simulink model "MPC"  (R2018a)
settings: Solver=VariableStepAuto  StartTime=0.0  StopTime=10  RelTol=1e-3
PreLoadFcn:
  | modelDir = fileparts(get_param(bdroot, 'FileName'));
  | addpath(modelDir);
  | addpath(fullfile(modelDir,'../../Parameters'));
  | addpath(fullfile(modelDir,'../../Controllers/MPC'));
  | addpath(fullfile(modelDir,'../../Controllers/MPC/functions'));
  | addpath(fullfile(modelDir,'../../Controllers/MPC/functions/polynomial'));
  | addpath(fullfile(modelDir,'../../Controllers/MPC/functions/trajectory'));
  | addpath(fullfile(modelDir,'../../Controllers/MPC/functions/visualization'));
  | addpath(fullfile(modelDir,'../../Controllers/MPC/generated'));
  | addpath(fullfile(modelDir,'../../Misc'));
  | 
  | Parameters_Controllers % for controller sample rate
  | Parameters_Simulation
  | Constants_Kugle
  | Constants_nominal
  | Parameters_MPC;
  | 
  | PrepareMPCtrajectory;
InitFcn:
  | Parameters_Controllers % for controller sample rate
  | Parameters_Simulation
  | Constants_Kugle
  | Constants_nominal
  | Parameters_MPC;
  | 
  | close all; % close opened plots to prepare for automatic plots for MPC visualization
  | 
  | PrepareMPCtrajectory;
values from neighbouring files (symbols this model uses):
  MPC_Obstacles = [MPC_Obstacles; repmat([100, 100, 1], [(5-size(MPC_Obstacles,1)),1])]    [PrepareMPCtrajectory.m]
undefined symbols (not defined in the file or in its folder): maxAngle, maxdOmegaRef, maxOmegaRef, maxVelocity, minVelocity, MPC_DesiredVelocity, MPC_HeadingAngularVelocity, MPC_Trajectory, MPC_u0, MPC_x0, N, pathApproximationOrder, ProximityOffset, ProximityScale, Ts, Ts_MPC, WindowHeight, WindowOffset, WindowOrientationSelection, WindowWidth, Wmat, WNmat, x_init
libraries: qlib x1
settings Model: Creator=Thomas  LastModifiedBy=Thomas
settings DataIOCC: SaveOutput=off  SignalLogging=off  DSMLogging=off
settings ModelReferenceCC: ModelReferenceNumInstancesAllowed=Single  ModelReferencePassRootInputsByReference=off  ModelReferenceMinAlgLoopOccurrences=on

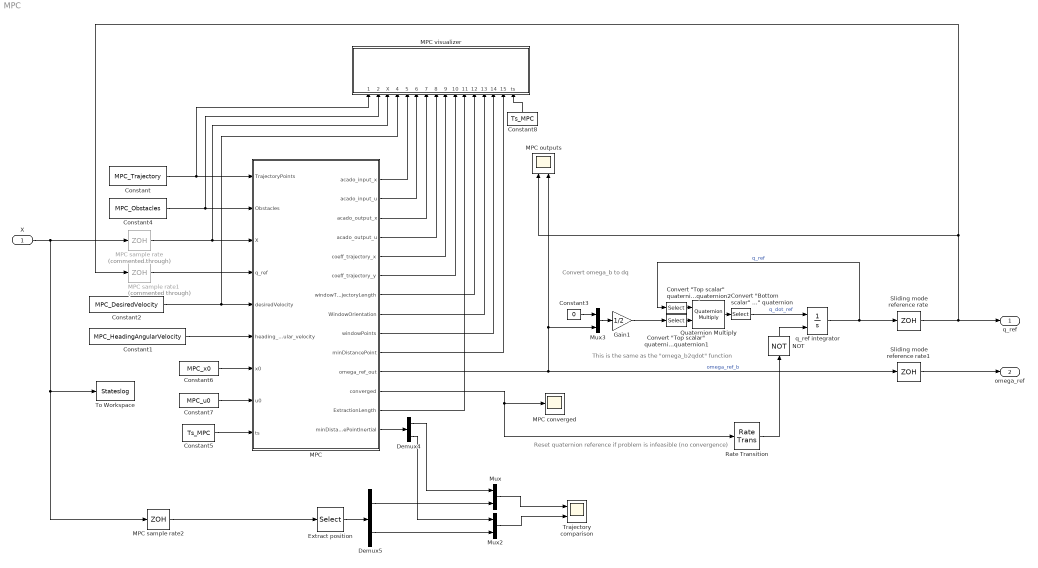
== system MPC ==
  note: Reset quaternion reference if problem is infeasible (no convergence)
  note: This is the same as the "omega_b2qdot" function
  note: Convert omega_b to dq
  X : Inport  PortDimensions=12
  Constant : Constant  Value=MPC_Trajectory  SampleTime=-1
  Constant1 : Constant  Value=MPC_HeadingAngularVelocity  SampleTime=-1
  Constant2 : Constant  Value=MPC_DesiredVelocity  SampleTime=-1
  Constant3 : Constant  Value=0
  Constant4 : Constant  Value=MPC_Obstacles  SampleTime=-1
  Constant5 : Constant  Value=Ts_MPC  SampleTime=-1
  Constant6 : Constant  Value=MPC_x0  SampleTime=-1
  Constant7 : Constant  Value=MPC_u0  SampleTime=-1
  Constant8 : Constant  Value=Ts_MPC  SampleTime=Ts_MPC
  "Convert \"Bottom scalar\" quaternion to \"Top scalar\" quaternion" : Selector  InputPortWidth=4  IndexOptions=Index vector (dialog)  Indices=[4 1 2 3]  OutputSizes=1
  "Convert \"Top scalar\" quaternion to \"Bottom scalar\" quaternion1" : Selector  InputPortWidth=4  IndexOptions=Index vector (dialog)  Indices=[2 3 4 1]  OutputSizes=1
  "Convert \"Top scalar\" quaternion to \"Bottom scalar\" quaternion2" : Selector  InputPortWidth=4  IndexOptions=Index vector (dialog)  Indices=[2 3 4 1]  OutputSizes=1
  Demux4 : Demux  Outputs=2
  Demux5 : Demux  Outputs=2
  Extract position : Selector  InputPortWidth=12  IndexOptions=Index vector (dialog)  Indices=[1 2]  OutputSizes=1
  Gain1 : Gain  Gain=1/2
  MPC : MATLAB Function  TreatAsAtomicUnit=on  SystemSampleTime=Ts_MPC
      settings: MinAlgLoopOccurrences=on
  MPC converged : Scope
  MPC outputs : Scope  NumInputPorts=2
  MPC sample rate : ZeroOrderHold  Commented=through  SampleTime=Ts_MPC
  MPC sample rate1 : ZeroOrderHold  Commented=through  SampleTime=Ts_MPC
  MPC sample rate2 : ZeroOrderHold  SampleTime=Ts_MPC
  MPC visualizer : MATLAB Function  TreatAsAtomicUnit=on  SystemSampleTime=Ts_MPC
      settings: MinAlgLoopOccurrences=on
  Mux : Mux  Inputs=2
  Mux2 : Mux  Inputs=2
  Mux3 : Mux  Inputs=2
  NOT : Logic  Operator=NOT  IconShape=distinctive  AllPortsSameDT=off  OutDataTypeStr=boolean
  Quaternion Multiply : qlib/Quaternion Multiply
  Rate Transition : RateTransition
  Sliding mode reference rate : ZeroOrderHold  SampleTime=Ts
  Sliding mode reference rate1 : ZeroOrderHold  SampleTime=Ts
  To Workspace : ToWorkspace  VariableName=Stateslog  SaveFormat=Timeseries  SampleTime=-1
  Trajectory comparison : Scope  NumInputPorts=2
  q_ref integrator : Integrator  ExternalReset=level hold  InitialCondition=x_init(3:6)
  q_ref : Outport  PortDimensions=4
  omega_ref : Outport  Port=2  PortDimensions=3
  wires:
  X/1 -> MPC sample rate/1, MPC sample rate2/1, To Workspace/1
  MPC/5(coeff_trajectory_x) -> MPC visualizer/9(coeff_trajectory_x)
  Constant2/1 -> MPC visualizer/4(velocity), MPC/5(desiredVelocity)
  Mux/1 -> Trajectory comparison/1
  MPC/10(minDistancePoint) -> MPC visualizer/15(minDistancePoint)
  MPC/14(minDistancePointInertial) -> Demux4/1
  Demux5/2 -> Mux2/2
  MPC/2(acado_input_u) -> MPC visualizer/6(acado_input_u)
  Demux5/1 -> Mux/2
  MPC sample rate/1 -> MPC visualizer/3(X), MPC/3(X)
  Mux2/1 -> Trajectory comparison/2
  Extract position/1 -> Demux5/1
  Demux4/2 -> Mux2/1
  MPC/6(coeff_trajectory_y) -> MPC visualizer/10(coeff_trajectory_y)
  Sliding mode reference rate/1 -> MPC sample rate1/1, MPC outputs/1, q_ref/1
  "Convert \"Bottom scalar\" quaternion to \"Top scalar\" quaternion"/1 -> q_ref integrator/1  "q_dot_ref"
  Demux4/1 -> Mux/1
  MPC sample rate1/1 -> MPC/4(q_ref)
  Constant/1 -> MPC visualizer/1(TrajectoryPoints), MPC/1(TrajectoryPoints)
  q_ref integrator/1 -> "Convert \"Top scalar\" quaternion to \"Bottom scalar\" quaternion2"/1, Sliding mode reference rate/1  "q_ref"
  MPC/1(acado_input_x) -> MPC visualizer/5(acado_input_x)
  MPC/8(WindowOrientation) -> MPC visualizer/13(WindowOrientation)
  MPC/4(acado_output_u) -> MPC visualizer/8(acado_output_u)
  MPC/3(acado_output_x) -> MPC visualizer/7(acado_output_x)
  MPC/7(windowTrajectoryLength) -> MPC visualizer/12(trajectoryLength)
  "Convert \"Top scalar\" quaternion to \"Bottom scalar\" quaternion1"/1 -> Quaternion Multiply/2
  Gain1/1 -> "Convert \"Top scalar\" quaternion to \"Bottom scalar\" quaternion1"/1
  "Convert \"Top scalar\" quaternion to \"Bottom scalar\" quaternion2"/1 -> Quaternion Multiply/1
  Mux3/1 -> Gain1/1
  Constant3/1 -> Mux3/1
  Quaternion Multiply/1 -> "Convert \"Bottom scalar\" quaternion to \"Top scalar\" quaternion"/1
  MPC/11(omega_ref_out) -> Sliding mode reference rate1/1, MPC outputs/2, Mux3/2  "omega_ref_b"
  Constant1/1 -> MPC/6(heading_angular_velocity)
  Constant5/1 -> MPC/9(ts)
  Constant4/1 -> MPC visualizer/2(Obstacles), MPC/2(Obstacles)
  Sliding mode reference rate1/1 -> omega_ref/1
  MPC sample rate2/1 -> Extract position/1
  Constant6/1 -> MPC/7(x0)
  Constant7/1 -> MPC/8(u0)
  MPC/13(ExtractionLength) -> MPC visualizer/11(ExtractionLength)
  Constant8/1 -> MPC visualizer/16(ts)
  MPC/9(windowPoints) -> MPC visualizer/14(windowPoints)
  NOT/1 -> q_ref integrator/2
  MPC/12(converged) -> Rate Transition/1, MPC converged/1
  Rate Transition/1 -> NOT/1

== matlab function MPC/MPC ==
  data: TrajectoryPoints input; Obstacles input; X input size=12; q_ref input size=4; desiredVelocity input; heading_angular_velocity input; N parameter; x0 input size=[1,length(MPC_x0)]; u0 input size=[1,length(MPC_u0)]; acado_input_x output size=[N+1,length(MPC_x0)]; acado_input_u output size=[N,length(MPC_u0)]; acado_output_x output size=[N+1,length(MPC_x0)]; acado_output_u output size=[N,length(MPC_u0)]; coeff_trajectory_x output size=[10,1]; coeff_trajectory_y output size=[10,1]; windowTrajectoryLength output; WindowOrientation output; windowPoints output size=[100,2]; minDistancePoint output; omega_ref_out output; converged output; ExtractionLength output; minDistancePointInertial output; pathApproximationOrder parameter; WindowOrientationSelection parameter; minVelocity parameter; maxOmegaRef parameter; maxAngle parameter; WNmat parameter; Wmat parameter; ts input; maxVelocity parameter; maxdOmegaRef parameter; ProximityOffset parameter; ProximityScale parameter
function [acado_input_x, acado_input_u, acado_output_x, acado_output_u, coeff_trajectory_x, coeff_trajectory_y, windowTrajectoryLength, WindowOrientation, windowPoints, minDistancePoint, omega_ref_out, converged, ExtractionLength, minDistancePointInertial] = MPC(TrajectoryPoints, Obstacles, X, q_ref, desiredVelocity, heading_angular_velocity, N, x0, u0, pathApproximationOrder, WindowOrientationSelection, minVelocity, maxOmegaRef, maxAngle, WNmat, Wmat, ts, maxVelocity, maxdOmegaRef, ProximityOffset, ProximityScale)
    Phi = @(q)[q(1) -q(2) -q(3) -q(4);     % for q o p = Phi(q) * p
              q(2) q(1)  -q(4) q(3);
              q(3) q(4)  q(1)  -q(2);
              q(4) -q(3) q(2)  q(1)];           
    Gamma = @(p)[p(1) -p(2) -p(3) -p(4);   % for q o p = Gamma(p) * q
                 p(2) p(1) p(4) -p(3);
                 p(3) -p(4) p(1) p(2);
                 p(4) p(3) -p(2) p(1)];  

    devec = [0,1,0,0;0,0,1,0;0,0,0,1]; % 'v' in notes
    vec = [0,0,0;1,0,0;0,1,0;0,0,1]; % '^' in notes
   
    x = X(1);
    y = X(2);
    q1 = X(3);
    q2 = X(4);
    q3 = X(5);
    q4 = X(6);
    q = [q1,q2,q3,q4]';
   
    % OBS! It seems to be quite important to use the filtered translational velocity which does not have spikes due to changes in the attitude
    dx = X(7);
    dy = X(8);
    dq1 = X(9);
    dq2 = X(10);
    dq3 = X(11);
    dq4 = X(12);      
        
    coder.extrinsic('ExtractWindowTrajectory_mex');
    coder.extrinsic('ExtractDistanceTrajectory_mex');
    coder.extrinsic('kugle_mpc_obstacles');
    
    % Convert states for MPC abstraction (robot-centric frame - Ferret frame???)      
    ResetAtConvergenceProblems = false;
    UseCurrentQuaternionAsReference = false; % if set to true, the current system state will be used at each iteration to define the current quaternion
    if (~UseCurrentQuaternionAsReference)
        q = q_ref;
    end    
    
    % Extract current robot yaw (heading)
    p = Phi(q)*Gamma(q)'*[0,1,0,0]';
    RobotYaw = atan2(p(3),p(2));   
    q_heading = [cos(RobotYaw/2);0;0;sin(RobotYaw/2)];
    q_tilt = Phi(q_heading)' * q; % tilt in heading frame    
    if (q_tilt(1) < 0)
        q_tilt = -q_tilt; % invert q_tilt to take shortest rotation
    end
    R_heading = [cos(RobotYaw), sin(RobotYaw);
                 -sin(RobotYaw), cos(RobotYaw)];                   
           
    persistent PreviousHorizonLength;
    if (isempty(PreviousHorizonLength))   
        PreviousHorizonLength = 0;
    end

    persistent xInit; 
    if (isempty(xInit))   
        fprintf('Initializing MPC\n');
        %xInit = zeros(N+1, length(x0));        
        xInit = repmat(x0, [(N+1),1]);
        %xInit(:,7) = ts * desiredVelocity * (0:N)'; % generate increasing S init values based on desired velocity
        %xInit(:,8) = repmat(desiredVelocity, [N+1, 1]); % set ds to desired velocity when initializing
    end    
    persistent uInit; 
    if (isempty(uInit))                   
        %uInit = zeros(N, length(u0));
        uInit = repmat(u0, [N,1]);
    end      
    
    ExtractionLength = 1.3*PreviousHorizonLength;
    if (ExtractionLength < 3.0)
        ExtractionLength = 3.0;
    end
        
    nTrajPoints = 0;    
    WindowTrajectory_tmp = [];
    coder.varsize('WindowTrajectory_tmp', [length(TrajectoryPoints) 2]);
    WindowOrientation = 0;
    %[WindowTrajectory_tmp, nTrajPoints, WindowOrientation] = ExtractWindowTrajectory_mex(TrajectoryPoints, [x,y], RobotYaw, [dx,dy], 1.1*N*ts*desiredVelocity, WindowWidth, WindowHeight, WindowOffset, OrientationParameter);    
    [WindowTrajectory_tmp, nTrajPoints, WindowOrientation] = ExtractDistanceTrajectory_mex(TrajectoryPoints, [x,y], RobotYaw, [dx,dy], ExtractionLength, WindowOrientationSelection);    
    WindowTrajectory = zeros(nTrajPoints, 2);
    WindowTrajectory = WindowTrajectory_tmp(1:nTrajPoints, 1:2); % extract only returned number of points  
    
    R_window = [cos(WindowOrientation), sin(WindowOrientation);
               -sin(WindowOrientation), cos(WindowOrientation)];  
    
    % Compute reference path polynomial
    [ReferencePoints, coeff_trajectory_x, coeff_trajectory_y, windowTrajectoryLength, s_minDistancePoint] = FitReferencePathPolynomial(WindowTrajectory, pathApproximationOrder, desiredVelocity, ts, N+1);
    
    % Compute coordinate on reference path closest to the robot
    minDistancePoint_x = EvaluatePolynomial(coeff_trajectory_x, s_minDistancePoint);
    minDistancePoint_y = EvaluatePolynomial(coeff_trajectory_y, s_minDistancePoint);
    minDistancePoint = [minDistancePoint_x,minDistancePoint_y];
    %FirstReferencePoint = R_window'*ReferencePoints(1,1:2)' + [x;y];  % rotate back to inertial frame since the reference point is in the robo-centric frame with Window orientation
    
    minDistancePointInertial = R_window'*minDistancePoint' + [x;y];  % rotate back to inertial frame since the reference point is in the robo-centric frame with Window orientation
    
    % Compute Tilt direction
    %tiltDirection = R_window * [0,1,0,0;0,0,1,0] * Phi(q)*Gamma(q)'*[0,0,0,1]';    
    q_tilt_inertial = Gamma(q_heading)' * q; % tilt in inertial frame
    if (q_tilt_inertial(1) < 0) % negate quaternion
        q_tilt_inertial = -q_tilt_inertial;
    end
    % Compute tilt in window
    q_tilt_window = R_window * q_tilt_inertial(2:3);    
    
    % Set current states as initial value to MPC and set reference trajectory
    % Convert quaternion from inertial frame into heading frame type of quaternion
    % Note that first column, xInit(:,1), is time
    % xInit = [q2,q3, x,y, dx,dy, s,ds, omega_ref_x,omega_ref_y]
    xInit(1,1) = q_tilt_window(1) + rand(1,1)/1000; % q2    (add some small noise, as the problem other seem to become infeasible sometimes?)
    xInit(1,2) = q_tilt_window(2) + rand(1,1)/1000; % q3
    xInit(:,3) = xInit(:,3) - xInit(1,3); % make xInit(1,4) = 0   (centering the robot in the prediction window)
    xInit(:,4) = xInit(:,4) - xInit(1,4); % make xInit(1,5) = 0   (centering the robot in the prediction window)    
    xInit(1,5:6) = R_window * [dx;dy] +  rand(2,1)/100; % OBS. Inertial frame velocity gets rotated into heading frame/window frame        
    xInit(:,7) = xInit(:,7) - xInit(1,7); % make xInit(1,8) = 0
    
    % Prepare online data vector with reference path polynomial coefficients
    coeff_x = [zeros(1,10-length(coeff_trajectory_x)), coeff_trajectory_x'];
    coeff_y = [zeros(1,10-length(coeff_trajectory_y)), coeff_trajectory_y'];
    
    % And extract/compute nearest obstacles
    NearestObstacles = GetNearestObstacles([x, y], Obstacles, 5);
    % Prepare obstacle list and convert to MPC frame
    obstacle1 = NearestObstacles(1,:) - [x, y, 0];
    obstacle2 = NearestObstacles(2,:) - [x, y, 0];
    obstacle3 = NearestObstacles(3,:) - [x, y, 0];
    obstacle4 = NearestObstacles(4,:) - [x, y, 0];
    obstacle5 = NearestObstacles(5,:) - [x, y, 0];    

    % Prepare online data matrix
    od0 = [desiredVelocity, maxVelocity, maxAngle, maxOmegaRef, maxdOmegaRef, windowTrajectoryLength, s_minDistancePoint, coeff_x, coeff_y, obstacle1, obstacle2, obstacle3, obstacle4, obstacle5, ProximityOffset, ProximityScale];                                  
    
    % Assemble acado_input struct
    acado_input_W = Wmat;
    acado_input_WN = WNmat;    
    acado_input_od = repmat(od0, [N+1,1]); % Online data
    acado_input_x = xInit;    
    acado_input_x0 = xInit(1,:);
    acado_input_u = uInit;    
    acado_input_y = zeros(N, 14);
    acado_input_yN = zeros(1, 9);
    acado_input = struct('W', acado_input_W, ...
                         'WN', acado_input_WN, ...
                         'od', acado_input_od, ...
                         'x', acado_input_x, ...
                         'x0', acado_input_x0, ...
                         'u', acado_input_u, ...
                         'y', acado_input_y, ...
                         'yN', acado_input_yN);                         

    % Prepare output struct to inform Simulink about output sizes    
    acado_info = struct('status', 0, 'cpuTime', 0.01, 'kktValue', 100.1, 'objValue', 1.01, 'QP_iter', 20, 'QP_violation', 0);
    acado_output = struct('info', acado_info, 'x', zeros(N+1,size(xInit,2)), 'u', zeros(N,size(uInit,2)));

    % Run the MPC solver    
    acado_output = kugle_mpc_obstacles(acado_input);
    %acado_output = feval('kugle_mpc_obstacles', acado_input);
                        
    fprintf('%2.2f\n%2.2f\n%2.2f\n%2.2f\n---------------\n', acado_output.info.kktValue, acado_output.info.objValue, acado_output.info.QP_iter, acado_output.info.QP_violation);      
    
    % Set control output and shift solution to be ready for next step
    % Set the initialization parameters for next iteration to be the current MPC solution     
    converged = (acado_output.info.status == 0); % converged?    
    %if (converged || ~ResetAtConvergenceProblems) 
        xInit = [acado_output.x(2:end,:); acado_output.x(end,:)]; % start from step 1 (not 0) in current MPC solution and repeat final state in the end
        uInit = [acado_output.u(2:end,:); zeros(1,size(acado_output.u,2))]; % start from step 1 (not 0) in current MPC solution and insert zeros in the end
    %end                  
    
    if (converged)        
        PreviousHorizonLength = acado_output.x(end,7);   
    end

    % Control output is given in Window frame
    % We thus need to convert the window frame angular velocity to body frame
    persistent omega_ref_I; 
    if (isempty(omega_ref_I))                   
        omega_ref_I = [0;0;0];
    end      
    %omega_ref_xy_W = acado_output.x(2,9:10)'; % omega_ref in window frame
    if (converged)
        omega_ref_I(1:2) = omega_ref_I(1:2) + acado_output.u(1,1:2)' * ts;
        %domeg_ref_input = acado_output.u(1,1:2)';                   
    else
        omega_ref_I(1:2) = zeros(2,1);
    end    
    
    omega_ref_I(3) = heading_angular_velocity;

%     % First we convert omega_ref_xy_W to omega_ref_xy_I
%     omega_ref_xy_I = R_window' * omega_ref_xy_W;      
%     
%     % Assemble omega_ref vector in inertial frame
%     omega_ref_I = [omega_ref_xy_I; heading_angular_velocity];
    
    % Next we convert to body frame, I_omega_ref_input to B_omega_ref_input
    omega_ref_B = devec * Phi(q)' * Gamma(q) * vec * omega_ref_I;
    
    % Set outputs
    omega_ref_out = omega_ref_I;        
    acado_output_x = acado_output.x;
    acado_output_u = acado_output.u;
    windowPoints = WindowTrajectory; % for output/visualization
end

== matlab function MPC/MPC visualizer ==
  data: TrajectoryPoints input; Obstacles input; X input; velocity input; acado_input_x input size=[N+1,length(MPC_x0)]; acado_input_u input size=[N,length(MPC_u0)]; acado_output_x input size=[N+1,length(MPC_x0)]; acado_output_u input size=[N,length(MPC_u0)]; coeff_trajectory_x input size=[10,1]; coeff_trajectory_y input size=[10,1]; ExtractionLength input; trajectoryLength input; WindowOrientation input; windowPoints input size=[100,2]; minDistancePoint input; N parameter; ts input; pathApproximationOrder parameter; WindowOrientationSelection parameter; WindowWidth parameter; WindowHeight parameter; WindowOffset parameter
function PlotMPC(TrajectoryPoints, Obstacles, X, velocity, acado_input_x, acado_input_u, acado_output_x, acado_output_u, coeff_trajectory_x, coeff_trajectory_y, ExtractionLength, trajectoryLength, WindowOrientation, windowPoints, minDistancePoint, N, ts, pathApproximationOrder, WindowOrientationSelection, WindowWidth, WindowHeight, WindowOffset)  %#codegen
    Phi = @(q)[q(1) -q(2) -q(3) -q(4);     % for q o p = Phi(q) * p
              q(2) q(1)  -q(4) q(3);
              q(3) q(4)  q(1)  -q(2);
              q(4) -q(3) q(2)  q(1)];           
    Gamma = @(p)[p(1) -p(2) -p(3) -p(4);   % for q o p = Gamma(p) * q
                 p(2) p(1) p(4) -p(3);
                 p(3) -p(4) p(1) p(2);
                 p(4) p(3) -p(2) p(1)];  

    devec = [0,1,0,0;0,0,1,0;0,0,0,1]; % 'v' in notes
    vec = [0,0,0;1,0,0;0,1,0;0,0,1]; % '^' in notes
   
    x = X(1);
    y = X(2);
    q1 = X(3);
    q2 = X(4);
    q3 = X(5);
    q4 = X(6);
    q = [q1,q2,q3,q4]';

    dx = X(7);
    dy = X(8);
    dq1 = X(9);
    dq2 = X(10);
    dq3 = X(11);
    dq4 = X(12);    
    dq = [dq1,dq2,dq3,dq4]';
    
    coder.extrinsic('ExtractWindowTrajectory_mex');    
    coder.extrinsic('ExtractDistanceTrajectory_mex');    
    
    % Compute robot yaw (heading)
    p = Phi(q)*Gamma(q)'*[0,1,0,0]';
    RobotYaw = atan2(p(3),p(2));   

    persistent fig1;
    persistent ax1;
    if (isempty(fig1))
        fig1 = figure;
        ax1 = axes;
    end
    persistent fig2;
    persistent ax2;
    if (isempty(fig2))
        fig2 = figure;
        ax2 = axes;
    end    
    
    cla(ax1);
    cla(ax2);  

    MPCtrajectory = acado_output_x(:,3:4);        
    MPCsRef = acado_output_x(:,7);
    MPCreferencePoints = [polyval(coeff_trajectory_x, MPCsRef), polyval(coeff_trajectory_y, MPCsRef)];    
    
%     nTrajPoints = 0;    
%     WindowTrajectory_tmp = [];
%     coder.varsize('WindowTrajectory_tmp', [length(TrajectoryPoints) 2]);
%     WindowOrientation2 = 0;    
%     %[WindowTrajectory_tmp, nTrajPoints, WindowOrientation2] = ExtractWindowTrajectory_mex(TrajectoryPoints, [x,y], RobotYaw, [dx,dy], 1.1*N*ts*velocity, WindowWidth, WindowHeight, WindowOffset, OrientationParameter);    
%     [WindowTrajectory_tmp, nTrajPoints, WindowOrientation2] = ExtractDistanceTrajectory_mex(TrajectoryPoints, [x,y], RobotYaw, [dx,dy], ExtractionLength, WindowOrientationSelection);    
%     WindowTrajectory = zeros(nTrajPoints, 2);
%     WindowTrajectory = WindowTrajectory_tmp(1:nTrajPoints, 1:2); % extract only returned number of points        
%     if (WindowOrientation ~= WindowOrientation2)
%         disp('Orientation does not match');        
%     end
    
    WindowTrajectory = windowPoints;
    
    R_window = [cos(WindowOrientation), sin(WindowOrientation);
                 -sin(WindowOrientation), cos(WindowOrientation)];    
    
    InertialWindowPoints = RotateTrajectory(windowPoints, -WindowOrientation) + repmat([x, y], [length(windowPoints),1]);
    InertialMPCreferencePoints = RotateTrajectory(MPCreferencePoints, -WindowOrientation) + repmat([x, y], [length(MPCreferencePoints),1]);
    InertialMPCtrajectory = RotateTrajectory(MPCtrajectory, -WindowOrientation) + repmat([x, y], [length(MPCtrajectory),1]);    
    InertialWindowTrajectory = RotateTrajectory(WindowTrajectory, -WindowOrientation) + repmat([x, y], [length(WindowTrajectory),1]);
    
    plot(ax1, TrajectoryPoints(:,1), TrajectoryPoints(:,2), 'k-', 'MarkerSize', 10);
    hold(ax1, 'on');   
    plot(ax1, InertialWindowTrajectory(:,1), InertialWindowTrajectory(:,2), 'k*', 'MarkerSize', 2);
    tiltDirectionGlobal = [0,1,0,0;0,0,1,0] * Phi(q)*Gamma(q)'*[0,0,0,1]';  % Compute Tilt direction  
    PlotAxRobotWithTiltAndVelocity(ax1, [x,y], RobotYaw, 0.05, [dx,dy], tiltDirectionGlobal');
    plot(ax1, InertialMPCreferencePoints(:,1), InertialMPCreferencePoints(:,2), 'go', 'MarkerSize', 3);
    plot(ax1, InertialMPCtrajectory(:,1), InertialMPCtrajectory(:,2), 'r*', 'MarkerSize', 3);  
%     WindowCornersCentered = [-WindowHeight/2, -WindowWidth/2
%                               WindowHeight/2, -WindowWidth/2
%                               WindowHeight/2, WindowWidth/2
%                               -WindowHeight/2, WindowWidth/2
%                               -WindowHeight/2, -WindowWidth/2] + repmat(WindowOffset, [5,1]);                     
%     WindowCorners = RotateTrajectory(WindowCornersCentered, -WindowOrientation) + repmat([x, y], [5,1]);
%     plot(ax1, WindowCorners(:,1), WindowCorners(:,2), 'k--');   
    % plot obstacles
    for (j = 1:size(Obstacles,1))
        d = 2 * Obstacles(j,3);
        px = Obstacles(j,1) - Obstacles(j,3);
        py = Obstacles(j,2) - Obstacles(j,3);
        rectangle(ax1, 'Position',[px py d d],'Curvature',[1,1],'EdgeColor',[0 0 1]);            
    end

    hold(ax1, 'off');    
    axis(ax1, 'equal');
    xlim(ax1, [min(TrajectoryPoints(:,1))*2, max(TrajectoryPoints(:,1))*2]);
    ylim(ax1, [min(TrajectoryPoints(:,2))*2, max(TrajectoryPoints(:,2))*2]);    
    
    plot(ax2, -WindowTrajectory(:,2), WindowTrajectory(:,1), 'k*'); % plot rotated
    hold(ax2, 'on');
    Vel = R_window * [dx;dy];       
    tiltDirection = R_window * [0,1,0,0;0,0,1,0] * Phi(q)*Gamma(q)'*[0,0,0,1]';  % Compute Tilt direction     
    PlotAxRobotWithTiltAndVelocity(ax2, [0,0], deg2rad(90)+RobotYaw-WindowOrientation, 0.05, [-Vel(2),Vel(1)], [-tiltDirection(2),tiltDirection(1)]);    
    if (trajectoryLength > 0) % plot trajectory
        s = (0:0.01:trajectoryLength)';
        trajectory_x = EvaluatePolynomial(coeff_trajectory_x, s);
        trajectory_y = EvaluatePolynomial(coeff_trajectory_y, s);
        plot(ax2, -trajectory_y, trajectory_x, 'b-');
    end    
    plot(ax2, -MPCreferencePoints(:,2), MPCreferencePoints(:,1), 'g*');
    plot(ax2, -MPCtrajectory(:,2), MPCtrajectory(:,1), 'r*');      
    % plot obstacle
    for (j = 1:size(Obstacles,1))
        d = 2 * Obstacles(j,3);
        px = -(Obstacles(j,2) - y) - Obstacles(j,3);
        py = (Obstacles(j,1) - x) - Obstacles(j,3);
        rectangle(ax2, 'Position',[px py d d],'Curvature',[1,1],'EdgeColor',[0 0 1]);            
    end       
    hold(ax2, 'off');
    axis(ax2, 'equal');
    xlim(ax2, [-WindowWidth/2 + WindowOffset(2), WindowWidth/2 + WindowOffset(2)]);
    ylim(ax2, [-WindowHeight/2 + WindowOffset(1), WindowHeight/2 + WindowOffset(1)]);    
    
    %legend(ax, 'Robot', 'Velocity vector', 'Tilt direction', 'Approximated evenly-space trajectory (MPC reference)', 'MPC trajectory');
    
end
